simulink model "untitled"  (R2016a)
settings: Solver=VariableStepAuto  StartTime=0.0  StopTime=25  RelTol=1e-3
settings Model: Creator=Student  LastModifiedBy=Student

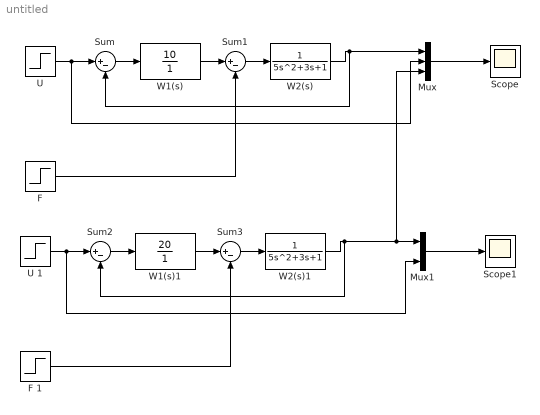
== system untitled ==
  "F " : Step  Time=0  SampleTime=0
  F 1 : Step  Time=0  SampleTime=0
  Mux : Mux  Inputs=3
  Mux1 : Mux  Inputs=2
  Scope : Scope
  Scope1 : Scope
  Sum{,1..3} (4 alike) : Sum  Inputs=|+-
  "U " : Step  Time=0  After=0  SampleTime=0
  U 1 : Step  Time=0  After=0  SampleTime=0
  W1(s) : TransferFcn  Numerator=[10]  Denominator=[1]
  W1(s)1 : TransferFcn  Numerator=[20]  Denominator=[1]
  W2(s) : TransferFcn  Denominator="[5  3  1]"
  W2(s)1 : TransferFcn  Denominator="[5  3  1]"
  wires:
  "U "/1 -> Mux/2, Sum/1
  W1(s)/1 -> Sum1/1
  Sum1/1 -> W2(s)/1
  Sum/1 -> W1(s)/1
  Mux/1 -> Scope/1
  "F "/1 -> Sum1/2
  W2(s)/1 -> Sum/2, Mux/1
  U 1/1 -> Mux1/2, Sum2/1
  W1(s)1/1 -> Sum3/1
  Sum3/1 -> W2(s)1/1
  Sum2/1 -> W1(s)1/1
  Mux1/1 -> Scope1/1
  F 1/1 -> Sum3/2
  W2(s)1/1 -> Sum2/2, Mux/3, Mux1/1
